simulink model "Lab1EE382"  (R2016a)
settings: Solver=VariableStepAuto  StartTime=0.0  StopTime=10.0  RelTol=1e-3
libraries: powerlib_meascontrol x2
settings Model: Creator=Tryrant  LastModifiedBy=Tryrant

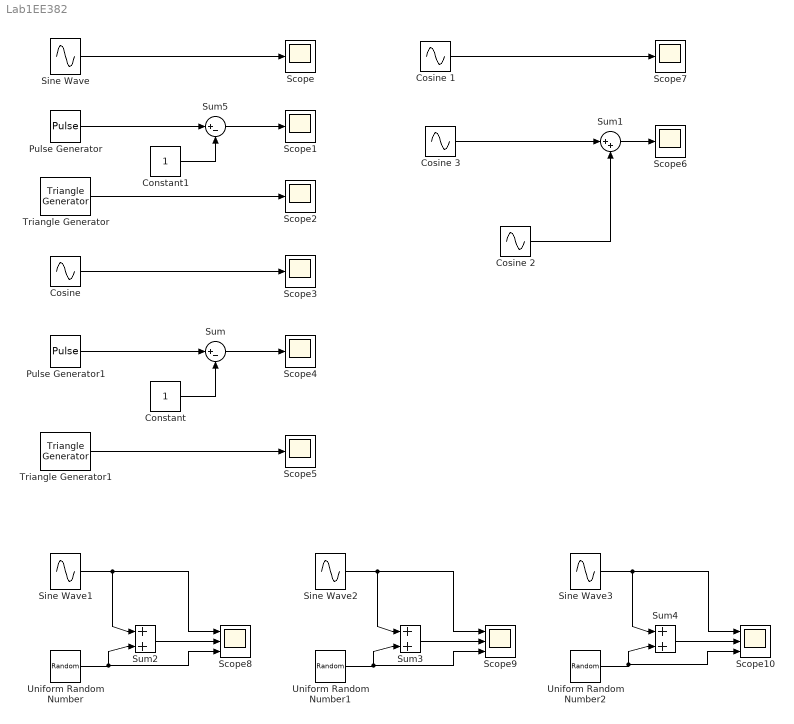
== system Lab1EE382 ==
  Constant : Constant
  Constant1 : Constant
  "Cosine " : Sin  Phase=pi/2  SampleTime=0
  Cosine 1 : Sin  Amplitude=5  Frequency=15  Phase=0.75*pi  SampleTime=0
  Cosine 2 : Sin  Amplitude=5  Frequency=10  Phase=0.8*pi  SampleTime=0
  Cosine 3 : Sin  Amplitude=5  Frequency=15  SampleTime=0
  Pulse Generator : DiscretePulseGenerator  PulseType=Time based  Amplitude=2  Period=4  PulseWidth=50  PhaseDelay=2
  Pulse Generator1 : DiscretePulseGenerator  PulseType=Time based  Amplitude=2  Period=4  PulseWidth=50  PhaseDelay=1
  Scope{,1..7} (8 alike) : Scope
  Scope10 : Scope  NumInputPorts=3
  Scope8 : Scope  NumInputPorts=3
  Scope9 : Scope  NumInputPorts=3
  Sine Wave : Sin  SampleTime=0
  Sine Wave1 : Sin  Amplitude=5  Frequency=10  SampleTime=0
  Sine Wave2 : Sin  Amplitude=2  Frequency=20  SampleTime=0
  Sine Wave3 : Sin  Amplitude=10  Frequency=50  SampleTime=0
  Sum : Sum  Inputs=|+-
  Sum1 : Sum  Inputs=|++
  Sum2 : Sum  Inputs=+||||+
  Sum3 : Sum  Inputs=+||||+
  Sum4 : Sum  Inputs=+||||+
  Sum5 : Sum  Inputs=|+-
  Triangle Generator : powerlib_meascontrol/Pulse & Signal Generators/Triangle Generator  Freq=1  Phase=90  Ts=0
  Triangle Generator1 : powerlib_meascontrol/Pulse & Signal Generators/Triangle Generator  Freq=1  Phase=0  Ts=0
  Uniform Random Number : UniformRandomNumber  Minimum=-1/2  Maximum=1/2  SampleTime=0.1
  Uniform Random Number1 : UniformRandomNumber  Minimum=-1/2  Maximum=1/2  SampleTime=0.1
  Uniform Random Number2 : UniformRandomNumber  Minimum=-1/2  Maximum=1/2  SampleTime=0.1
  wires:
  "Cosine "/1 -> Scope3/1
  Triangle Generator/1 -> Scope2/1
  Triangle Generator1/1 -> Scope5/1
  Sine Wave/1 -> Scope/1
  Pulse Generator1/1 -> Sum/1
  Constant/1 -> Sum/2
  Sum/1 -> Scope4/1
  Cosine 1/1 -> Scope7/1
  Sum1/1 -> Scope6/1
  Cosine 2/1 -> Sum1/2
  Cosine 3/1 -> Sum1/1
  Sum2/1 -> Scope8/2
  Sine Wave1/1 -> Scope8/1, Sum2/1
  Uniform Random Number/1 -> Scope8/3, Sum2/2
  Sum3/1 -> Scope9/2
  Sine Wave2/1 -> Scope9/1, Sum3/1
  Uniform Random Number1/1 -> Scope9/3, Sum3/2
  Sine Wave3/1 -> Scope10/1, Sum4/1
  Uniform Random Number2/1 -> Scope10/3, Sum4/2
  Pulse Generator/1 -> Sum5/1
  Constant1/1 -> Sum5/2
  Sum5/1 -> Scope1/1
  Sum4/1 -> Scope10/2
